simulink model "Hw2_sim"  (R2021a)
settings: Solver=VariableStepAuto  StartTime=0.0  StopTime=5.4  RelTol=1e-3
values from neighbouring files (symbols this model uses):
  A = [0 1;-3 -2]    [hw2.m]
  B = [0;1]    [hw2.m]
  C = [1 1]    [hw2.m]
  G = expm(A*Ts)    [hw2.m]
  tau0 = (G^(1/3)-eye(2))/A*B    [hw2.m]
  tau1 = (G-G^(1/3))/A*B    [hw2.m]
libraries: cstblocks x1
settings Model: Creator=paul8  LastModifiedBy=paul8

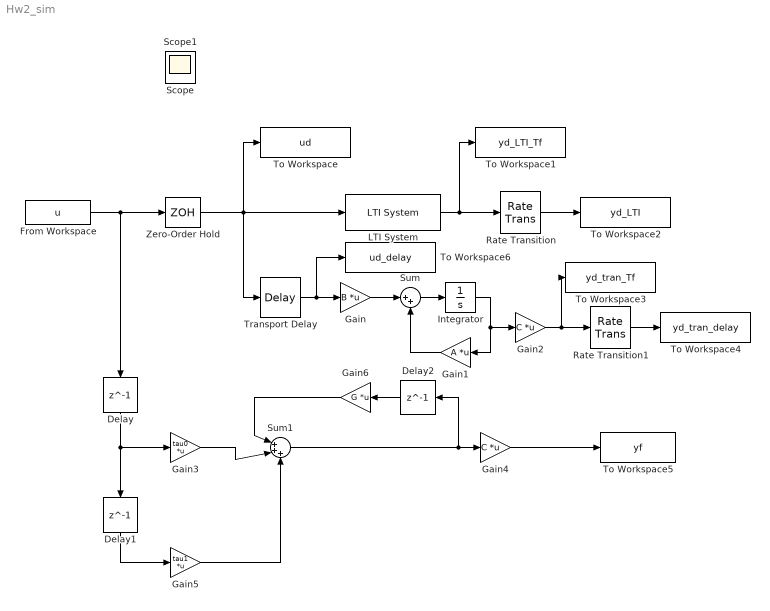
== system Hw2_sim ==
  Delay : Delay  DelayLength=1  InitialCondition=0  InputProcessing=Columns as channels (frame based)  UseCircularBuffer=on  SampleTime=0.18
  Delay1 : Delay  DelayLength=1  InitialCondition=0  InputProcessing=Columns as channels (frame based)  SampleTime=0.18
  Delay2 : Delay  DelayLength=1  InitialCondition=0  SampleTime=0.18
  From Workspace : FromWorkspace  VariableName=u  SampleTime=-1
  Gain : Gain  Gain=B  Multiplication=Matrix(K*u)
  Gain1 : Gain  Gain=A  Multiplication=Matrix(K*u)
  Gain2 : Gain  Gain=C  Multiplication=Matrix(K*u)
  Gain3 : Gain  Gain=tau0  Multiplication=Matrix(K*u)
  Gain4 : Gain  Gain=C  Multiplication=Matrix(K*u)
  Gain5 : Gain  Gain=tau1  Multiplication=Matrix(K*u)
  Gain6 : Gain  Gain=G  Multiplication=Matrix(K*u)
  Integrator : Integrator
  LTI System : cstblocks/LTI System  sys=sys  IC=[]
  Rate Transition : RateTransition  OutPortSampleTime=0.18
  Rate Transition1 : RateTransition  OutPortSampleTime=0.18
  Sum : Sum  Inputs=|++
  Sum1 : Sum  Inputs=|+++
  To Workspace : ToWorkspace  VariableName=ud  SampleTime=0.06
      settings: Save2DSignal=2-D array (concatenate along first dimension)
  To Workspace1 : ToWorkspace  VariableName=yd_LTI_Tf  SampleTime=0.06
  To Workspace2 : ToWorkspace  VariableName=yd_LTI  SampleTime=0.18
  To Workspace3 : ToWorkspace  VariableName=yd_tran_Tf  SampleTime=0.06
  To Workspace4 : ToWorkspace  VariableName=yd_tran_delay  SampleTime=0.18
  To Workspace5 : ToWorkspace  VariableName=yf  SampleTime=0.18
  To Workspace6 : ToWorkspace  VariableName=ud_delay  SampleTime=0.06
  Transport Delay : TransportDelay  DelayTime=0.12
  Zero-Order Hold : ZeroOrderHold  SampleTime=0.18
  Scope : Scope
  Scope1 : Scope
  wires:
  From Workspace/1 -> Zero-Order Hold/1, Delay/1
  Zero-Order Hold/1 -> LTI System/1, Transport Delay/1, To Workspace/1
  LTI System/1 -> To Workspace1/1, Rate Transition/1
  Rate Transition/1 -> To Workspace2/1
  Transport Delay/1 -> To Workspace6/1, Gain/1
  Gain/1 -> Sum/1
  Sum/1 -> Integrator/1
  Integrator/1 -> Gain2/1, Gain1/1
  Gain1/1 -> Sum/2
  Gain2/1 -> To Workspace3/1, Rate Transition1/1
  Rate Transition1/1 -> To Workspace4/1
  Delay/1 -> Gain3/1, Delay1/1
  Delay1/1 -> Gain5/1
  Gain5/1 -> Sum1/3
  Gain3/1 -> Sum1/2
  Sum1/1 -> Delay2/1, Gain4/1
  Delay2/1 -> Gain6/1
  Gain6/1 -> Sum1/1
  Gain4/1 -> To Workspace5/1
